simulink model "c2000_host_solar"  (R2021b)
settings: Solver=VariableStepAuto  StartTime=0.0  StopTime=inf  RelTol=1e-3
InitFcn:
  | run('Solar_Inverter.m');
values from neighbouring files (symbols this model uses):
  P_Value = [0.200000000000000,7.20500000000000;0.300000000000000,10.8100000000000;0.400000000000000,14.4100000000000;0.500000000000000,18.0100000000000;0.600000000000000,21.6100000000000;0.700000000000000,25.2200000000000;0.800000000000000,28.8200000000000;0.900000000000000,32.4200000000000;1,36.0200000000000]    [Solar_Inverter.m]
libraries: instrumentseriallib x3, demo_controls x1, simulink x1
CloseFcn:
  | clear PV_Current PV_Voltage Ts1 Ts2 Tc1 Tc2 P_Value;
settings Model: Creator=The MathWorks, Inc.  LastModifiedBy=The MathWorks, Inc.
settings SolverCC: AlgebraicLoopSolver=TrustRegion
settings DataIOCC: SaveOutput=off  SaveTime=off  ReturnWorkspaceOutputs=off
settings DebuggingCC: ParameterPrecisionLossMsg=none  SFMachineParentedDataDiag=warning  ArithmeticOperatorsInVariantConditions=warning
settings SFSimCC: SimUseLocalCustomCode=off  CustomCodeUndefinedFunction=UseInterfaceOnly
settings RTWCC: RTWUseLocalCustomCode=off

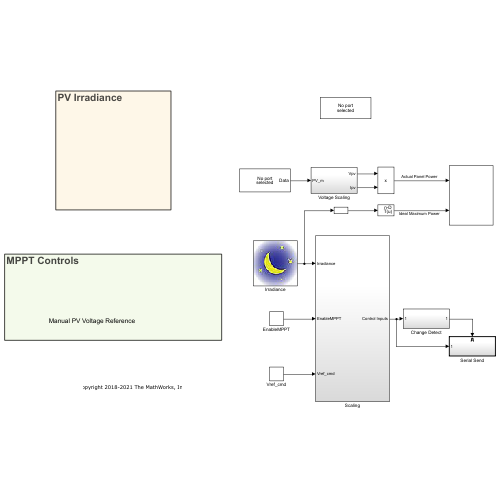
[thumbnail: Simulink's stored preview of the top-level diagram]
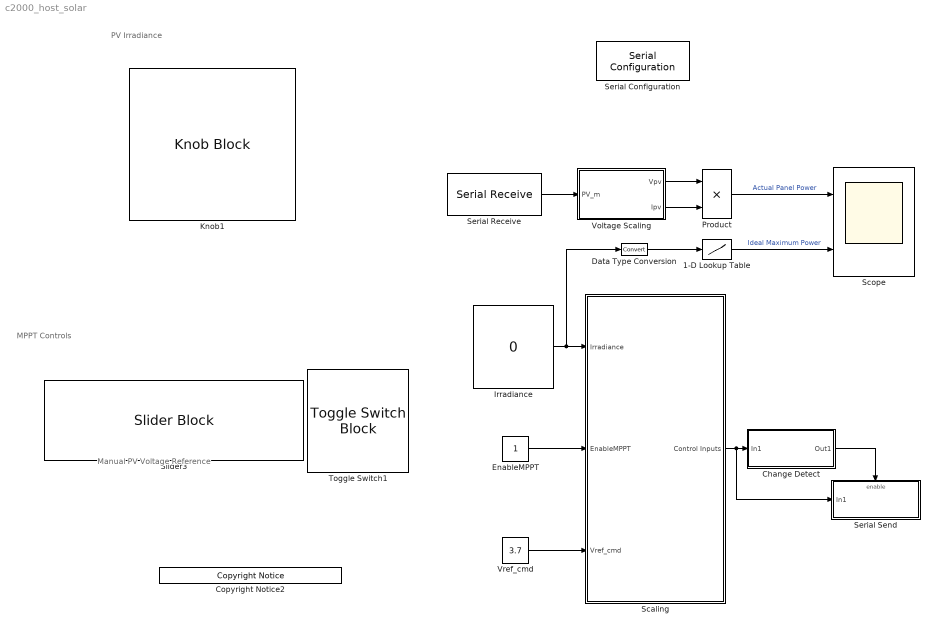
== system c2000_host_solar ==
  note: MPPT Controls
  note: PV Irradiance
  note: Manual PV Voltage Reference
  1-D Lookup Table : Lookup_n-D  NumberOfTableDimensions=1  BreakpointsForDimension1=P_Value(:,1)  Table=P_Value(:,2)  InternalRulePriority=Speed  RndMeth=Simplest  InputSameDT=on
  Change Detect : Subsystem
  Copyright Notice2 : demo_controls/Copyright Notice  year=2018  prod=tic2000
      settings: SourceProductBaseCode=ME
  Data Type Conversion : DataTypeConversion
  EnableMPPT : Constant  OutDataTypeStr=single
  Irradiance : Constant  Value=0  OutDataTypeStr=fixdt(1,32,13)  SampleTime=0.05
      mask Display:
      | I = str2double(get_param(gcb,'Value'));
      | ud = get_param(gcb,'UserData');
      | if(I < 0.2)
      |     image(ud.im1);
      | elseif(I >= 0.2 && I < 0.4)
      |     image(ud.im2);
      | elseif(I >= 0.4 && I < 0.6)
      |     image(ud.im3);
      | else
      |     image(ud.im4);
      | end
  Knob1 : KnobBlock  ScaleMax=0.80000000000000004  TickInterval=0.10000000000000001
  Product : Product
  Scaling : Subsystem
  Scope : Scope  NumInputPorts=2
  Serial Configuration : instrumentseriallib/Serial Configuration  Priority=-200000  Port=<Select a port...>  ComPort=<Select a port...>  BaudRate=1500000  DataBits=8  Parity=none  StopBits=1  ByteOrder=little-endian  FlowControl=none  Timeout=10  SimulateUsing=Interpreted execution  BlockInModel=on
  Serial Receive : instrumentseriallib/Serial Receive  Port=<Select a port...>  ComPort=COM9  DataType=uint16  SaveDataType=uint8  ToggleHeader=on  Header="[ 83  83 ]"  ToggleTerminator=on  Terminator=Custom terminator  CustomTerminator="[ 69  69 ]"  ToggleDataSize=on  DataSize="[2  10]"  EnableBlockingMode=on  ActionDataUnavailable=Output last received value  ActionWhenDataUnavailable=Output last received value  CustomValue=2  SampleTime=0.05  SimulateUsing=Interpreted execution  BlockInModel=on
  Serial Send : Subsystem  TreatAsAtomicUnit=on
  Slider3 : SliderBlock  ScaleMin=1  ScaleMax=10  TickInterval=1
  Toggle Switch1 : ToggleSwitchBlock  LabelPosition=Hide
      settings: Values={{'Manual Vref', 'Enable MPPT'}, [0 1]}
  Voltage Scaling : Subsystem
  Vref_cmd : Constant  Value=3.7  OutDataTypeStr=single
  wires:
  Voltage Scaling/2(Ipv) -> Product/2
  Voltage Scaling/1(Vpv) -> Product/1
  Change Detect/1(Out1) -> Serial Send/Enable
  Product/1 -> Scope/1  "Actual Panel Power"
  1-D Lookup Table/1 -> Scope/2  "Ideal Maximum Power"
  Data Type Conversion/1 -> 1-D Lookup Table/1
  Irradiance/1 -> Data Type Conversion/1, Scaling/1(Irradiance)
  EnableMPPT/1 -> Scaling/2(EnableMPPT)
  Vref_cmd/1 -> Scaling/3(Vref_cmd)
  Scaling/1(Control Inputs) -> Serial Send/1(In1), Change Detect/1(In1)
  Serial Receive/1 -> Voltage Scaling/1(PV_m)

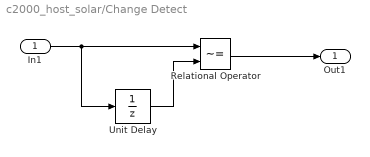
== system c2000_host_solar/Change Detect ==
  In1 : Inport
  Relational Operator : RelationalOperator  Operator=~=  OutDataTypeStr=boolean  RndMeth=Simplest
  Unit Delay : UnitDelay  SampleTime=-1  HasFrameUpgradeWarning=on
  Out1 : Outport  VectorParamsAs1DForOutWhenUnconnected=off
  wires:
  In1/1 -> Relational Operator/1, Unit Delay/1
  Unit Delay/1 -> Relational Operator/2
  Relational Operator/1 -> Out1/1

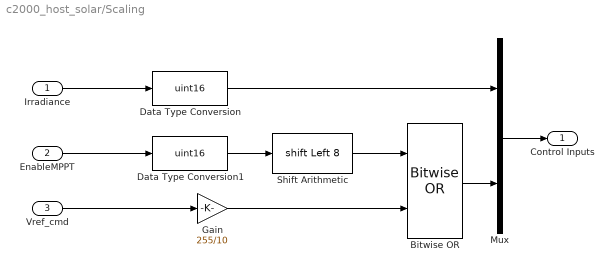
== system c2000_host_solar/Scaling ==
  Irradiance : Inport
  EnableMPPT : Inport  Port=2
  Vref_cmd : Inport  Port=3
  Bitwise OR : simulink/Logic and Bit Operations/Bitwise Operator  logicop=OR  UseBitMask=off  NumInputPorts=2  BitMask=bin2dec('11011001')  BitMaskRealWorld=Stored Integer
  Data Type Conversion : DataTypeConversion  OutDataTypeStr=uint16  ConvertRealWorld=Stored Integer (SI)
  Data Type Conversion1 : DataTypeConversion  OutDataTypeStr=uint16
  Gain : Gain  Gain=255/10  OutDataTypeStr=uint16
  Mux : Mux  Inputs=2
  Shift Arithmetic : ArithShift  BitShiftNumber=8  BitShiftDirection=Left
  Control Inputs : Outport  VectorParamsAs1DForOutWhenUnconnected=off
  wires:
  Irradiance/1 -> Data Type Conversion/1
  Vref_cmd/1 -> Gain/1
  EnableMPPT/1 -> Data Type Conversion1/1
  Data Type Conversion1/1 -> Shift Arithmetic/1
  Data Type Conversion/1 -> Mux/1
  Shift Arithmetic/1 -> Bitwise OR/1
  Gain/1 -> Bitwise OR/2
  Bitwise OR/1 -> Mux/2
  Mux/1 -> Control Inputs/1

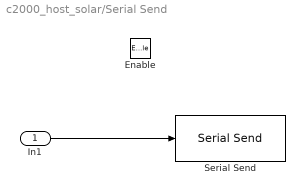
== system c2000_host_solar/Serial Send ==
  In1 : Inport
  Enable : EnablePort
  Serial Send : instrumentseriallib/Serial Send  Port=<Select a port...>  ComPort=COM9  Header=[]  Terminator=<none>  CustomTerminator=[]  EnableBlockingMode=off  SimulateUsing=Interpreted execution  BlockInModel=on
  wires:
  In1/1 -> Serial Send/1

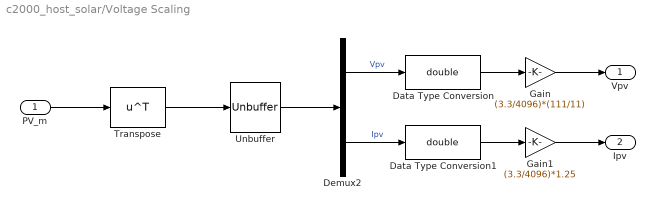
== system c2000_host_solar/Voltage Scaling ==
  PV_m : Inport
  Data Type Conversion : DataTypeConversion  OutDataTypeStr=double
  Data Type Conversion1 : DataTypeConversion  OutDataTypeStr=double
  Demux2 : Demux  Outputs=2
  Gain : Gain  Gain=(3.3/4096)*(111/11)
  Gain1 : Gain  Gain=(3.3/4096)*1.25
  Transpose : Math  Operator=transpose  SignedPower=on  SaturateOnIntegerOverflow=on
  Unbuffer : Unbuffer
  Vpv : Outport  VectorParamsAs1DForOutWhenUnconnected=off
  Ipv : Outport  Port=2  VectorParamsAs1DForOutWhenUnconnected=off
  wires:
  Data Type Conversion/1 -> Gain/1
  Gain1/1 -> Ipv/1
  Data Type Conversion1/1 -> Gain1/1
  Gain/1 -> Vpv/1
  Transpose/1 -> Unbuffer/1
  PV_m/1 -> Transpose/1
  Unbuffer/1 -> Demux2/1
  Demux2/1 -> Data Type Conversion/1  "Vpv"
  Demux2/2 -> Data Type Conversion1/1  "Ipv"
